simulink model "changq_m"  (Simulink 7.9)
settings: Solver=ode45  SolverMode=SingleTasking  StartTime=0.0  StopTime=999999  MaxStep=10  RelTol=1e-3  AbsTol=1e-3
values from neighbouring files (symbols this model uses):
  U = st_Varia('LongNames')    [changq_i.m]
  x0 = []    [changq_i.m]    (also in changq_s.m = x0)
undefined symbols (not defined in the file or in its folder): B
settings Model: Creator=M.Sparnaaij  LastModifiedBy=M.Sparnaaij
settings DataIOCC: LimitDataPoints=off  SaveOutput=off  SaveTime=off  SignalLoggingName=sigsOut
settings OptimizationCC: BooleanDataType=off
settings DebuggingCC: SaveWithParameterizedLinksMsg=none  SignalResolutionControl=TryResolveAllWithWarning  SolverPrmCheckMsg=none  MultiTaskDSMMsg=warning  MultiTaskCondExecSysMsg=none  StrictBusMsg=None
settings HardwareCC: TargetUnknown=on
settings RTWCC: IncludeERTFirstTime=on
settings GRTTargetCC: CombineOutputUpdateFcns=off  GRTInterface=on

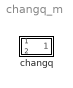
== system changq_m ==
  changq : Subsystem  Description=changq
      mask init:
      | filenaam='.\StimelaData\changq_p.mat';
      | 
      | [Pn,Fn,Fext]=Fileprop(filenaam);
      | 
      | errstr = st_UniqName(filenaam,'filenaam=''','SubSystem','OpenFcn');
      | if errstr, error([errstr 'The filename "' filenaam '" is already in use. Choose a different filename.']), end
      | 
      | P = changq_p(filenaam);
      | [B,x0,U]=changq_i(filenaam);
      settings: OpenFcn=|
      | filenaam='.\StimelaData\changq_p.mat';
      | st_ParameterInput('init',gcb,filenaam,'changq');
      mask Display:
      | plot(0,0,100,100,[0 20],[15 15],[0 20],[80 80],[0 20],[85 85],[80 100],[ 50 50],[80 100],[ 55 55]);
      | plot([20 80 80 20 20],[10 10 90  90 10])
      | text(50,50,'S', 'horizontalAlignment', 'center', 'verticalAlignment', 'middle');
      | disp('')

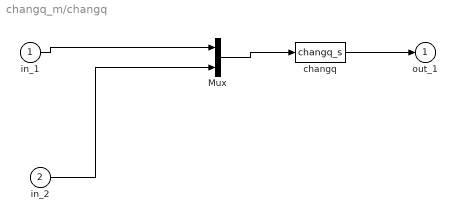
== system changq_m/changq ==
  in_1 : Inport
  in_2 : Inport  Port=2
  Mux : Mux  Inputs=2
  changq : S-Function  FunctionName=changq_s  Parameters=B,x0,U,P  EnableBusSupport=off
  out_1 : Outport  InitialOutput=0
  wires:
  changq/1 -> out_1/1
  in_1/1 -> Mux/1
  Mux/1 -> changq/1
  in_2/1 -> Mux/2
